simulink model "Copy_of_CM13_2024a_MachE_for_UA_HIL"  (R2024a)
settings: Solver=ode1  StartTime=0.0  StopTime=Inf  FixedStep=0.001  RelTol=1e-3  EnableMultiTasking=on
PreLoadFcn:
  | % if ~length(which('cmcmd')), cmenv; end
PostLoadFcn:
  | if any(exist('dsrtsu_mdlpostloadfcn', 'file') ~= 0), dsrtsu_mdlpostloadfcn('Execute', bdroot); end
InitFcn:
  | , if any(exist('rtifpga_mdlclblib', 'file') ~= 0), rtifpga_mdlclblib('Init', bdroot); end,
  | , if any(exist('dsmpb_private', 'file') ~= 0), dsmpb_private('dsmpb_mdlclblib', 'Init', bdroot); end,
undefined symbols (not defined in the file or in its folder): AccelCmd, ActTqLF_Nm_, ActTqLR_Nm_, ActTqRF_Nm_, ActTqRR_Nm_, BattChargeLimitMaxPwr, BattChargeLimitSocBpts, BattChargeLimitTbl, BattChrgCapcty, BattDischargeLimitSocBpts, BattDischargeLimitTbl, BattDischargeMaxPwr, BattNumCellsParallel, BattNumCellsSeries, BattOpenVoltCapBpts, BattOpenVoltTbl, BattResistSocBpts, BattResistTbl, BattResistTempBpts, BrakeMaxPrs, BrakeMaxTrq, ChassisDistCg2FrontAxle, ChassisDistCg2RearAxle, ChassisVehMass, CltchCmd, CoastDown, DecelCmd, DiffRatio, DiscIntNeverNeededParam, EnvGravCnst, EnvPrs, EnvTemp, FuelSpecificGrav, GearCmd, h, InitStates, lgSw, limitedMCT, MCT, MtrEffSpdBpts, MtrEffTbl, MtrEffTrqBpts, MtrPwrMax, MtrTrqMax, planned_speed, planned_time, pMCT, RealSimPara, ref_speed, Ref_speed, ref_time, Ref_time, rticanmm_blockfcn, rticanmm_initfcn, SteeringCmd, SupvsryCtrlRegenBrkCutOffTbl, SupvsryCtrlRegenSpdBpts, TestScnrioCycleNum, US06, VEH
libraries: simulink x264, VSIGenLib x262, etargetslib x201, dsmpblib x161, CarMaker4SL x142, rtimmsu_dsrtlib x32, vehdynlibtire x24, autolibshared x19, vehdynlibsuspension x14, vehdynlibtirecommon x14, autolibutils x10, VsrLibWheel x8
(part 9 of 47)

== system Copy_of_CM13_2024a_MachE_for_UA_HIL/CarMaker_new/IPG Vehicle/MachE CAN ==
  note: Working in Progress
  note: Gear_Shift_By_Wire_3_HS1
      | TrnGear_D_RqPt
      |
      | No_Gear
      | 0
      |
      | Park
      | 1
      |
      | Reverse
      | 2
      |
      | Neutral
      | 3
      |
      | Drive
      | 4
      |
      | Manual
      | 5
      |
      | NotUsed
      | 6
      |
      | Fault
      | 7
  note: Gear_Shift_By_Wire_HS1
      | TrnGear_D_RqDrv
      |
      | No_Gear
      | 0
      |
      | Park
      | 1
      |
      | Reverse
      | 2
      |
      | Neutral
      | 4
      |
      | Drive
      | 8
      |
      | Manual
      | 16
      |
      | Return_To_Park
      | 21/26
      |
      | Fault
      | 31
  Bus Creator : BusCreator  Inputs=6
  Bus Creator1 : BusCreator  Inputs=8
  Bus Selector : BusSelector  Commented=on  OutputSignals=Battery_Traction_2.BattTrac_U2_Actl,Battery_Traction_2.BattTrac_I2_Actl,PowertrainData_10_HS1.GearPos_D_Actl,PowertrainData_10_HS1.GearLvr_D_ActlDrv
  Bus Selector1 : BusSelector  OutputSignals=Accel_Data.VehLatLongVert_No_Cnt,Accel_Data.VehLatLongVertA_No_Cs,Accel_Data.VehVert2_A_Actl,Accel_Data.VehVertAActl_D_Qf,Accel_Data.VehLong2_A_Actl,Accel_Data.VehLongAActl_D_Qf,Accel_Data.VehLat2_A_Actl,Accel_Data.VehLatAActl_D_Qf,Yaw_Data.VehYawWActl_D_Qf,Yaw_Data.VehRolWActl_D_Qf,Yaw_Data.VehRollYaw_No_Cnt,Yaw_Data.VehRollYawW_No_Cs,Yaw_Data.VehYaw_W_Actl,Yaw_Data.VehRol_W_Actl
  Bus Selector2 : BusSelector  OutputSignals=VehLat2_A_Actl,VehLong2_A_Actl,VehVert2_A_Actl
  Bus Selector3 : BusSelector  OutputSignals=VehRol_W_Actl,VehYaw_W_Actl
  Bus Selector4 : BusSelector  OutputSignals=SteeringPinion_Data_HS2.StePinRelInit_An_Sns
  Constant : Constant  OutDataTypeStr=Inherit: Inherit via back propagation
  Constant1 : Constant  Value=0
  Gain{,1..2,6} (4 alike) : Gain  Commented=on
  Gain3 : Gain
  Gain4 : Gain
  Gain5 : Gain
  Multiport Switch : MultiPortSwitch  DataPortOrder=Zero-based contiguous  Inputs=2  zeroidx=on  SaturateOnIntegerOverflow=off  InputSameDT=off
  Multiport Switch1 : MultiPortSwitch  DataPortOrder=Zero-based contiguous  Inputs=2  zeroidx=on  SaturateOnIntegerOverflow=off  InputSameDT=off
  RTICANMM Gateway : Subsystem  InitFcn=rticanmm_initfcn(gcb, 'CANnedyGateway')  ClipboardFcn=rticanmm_blockfcn('ClipboardFcn', 'CANnedyGateway', gcb)  mask(RTICANMM){DSProperties=struct('RTI',struct('Version',uint32(1),'BlockType',struct('isSLSource',uint8(1),'isSLSink',uint8(1),'isHWSource',uint8(0),'isHWSink',uint8(0),'isSetup',uint8(0),'isInline',uint8(1),'isNonInline',uint8(0),'isInterrupt',uint8(0),'isChannelwise',uint8(0)),'IOBoardType','RTICANMM','UnitType','RTICANMM','Identifier','GATEWAY','DialogType','SL','BlockSet','RTICANMM','SlaveProcessor','CAN')), CANMMBlock=RCM_ECU, CANMMDestFolder=RTICANMM_FILES, CANMMDestBlock=RCM_Harness, CANMMProperties=struct('generaloptions',struct('gwdirection',1,'mainblksorsetups',0,'trchierarchie','','gatewayname','RCM_Gateway','mergetrc',1,'trcinclude',1,'ssOpts',struct('ssSetSampleTime','INHERITED_SAMPLE_TIME','ssSetOffsetTime','FIXED_IN_MINOR_STEP_OFFSET'),'j1939_sort_key','dir','olddirection',0),'CANGatewayID',1,'direction',struct('link',{'RCM_ECU','RCM_Harness'},'link_dbc_override',{0,0},'filesupport',{1,1},'usedirection',{true,true},'changeexcludeonline',{0,0},'excludelist',{struct('ids',{{'146','145'}},'idFormat',{{0,0}}),struct('ids',{{}},'idFormat',{{}})},'j1939',{0,0},'excludelist_j1939',{struct('id',{{}},'prio',{{}},'pdu_f',{{}},'pdu_s',{{}},'src',{{}}),struct('id',{{}},'prio',{{}},'pdu_f',{{}},'pdu_s',{{}},'src',{{}})},'data',{struct('Board','','BoardNum','','ChannelNum',''),struct('Board','','BoardNum','','ChannelNum','')},'database',{struct('FileName','RTICANMM_FILES\HS2_CAN_CX727_BEV_MY21_DCV_V21.dbc','IsRelative',1,'ClusterId',1,'ClusterList',{{'default'}}),struct('FileName','RTICANMM_FILES\HS2_CAN_CX727_BEV_MY21_DCV_V21.dbc','IsRelative',1,'ClusterId',1,'ClusterList',{{'default'}})},'FileName',{'',''},'IsRelative',{1,1},'ClusterId',{1,1},'ClusterList',{{'default'},{'default'}},'idlist',{[],[]}),'excludelist_j1939',struct('dbcsource',[],'id',{{}},'prio',{{}},'pdu_f',{{}},'pdu_s',{{}},'src',{{}}),'BlockDataVersion','4.0','directions',struct('setup',struct('source','TRC','logic','-','defaultTrc','ENABLE'),'enablematrix',struct('Direction',{['CAN Bus 1 <=> CAN Bus 2'],['CAN Bus 1  => CAN Bus 2'],['CAN Bus 1 <=  CAN Bus 2'],['CAN Bus 1  => CAN Bus 2'],['CAN Bus 1 <=  CAN Bus 2']},'Source',{'BOTH','NONE','NONE','BOTH','BOTH'},'Logic',{'OR','-','-','OR','OR'},'DefaultTrc',{'ENABLE','-','-','ENABLE','ENABLE'})),'blk',['HIL_MachE_CM10/Vehicle Under Test/Vehicle/MachE CAN/RTICANMM' char(10) 'Gateway'],'CANMMName','RCM_Gateway','TRC',struct('Name','RTICANMM_GW_RCM_Gateway_usr.trc','Path','C:\GitDev\Yunli\FordMachE\HIL-Operation\src_cm4sl\RTICANMM_FILES\RTICANMM_GW_RCM_Gateway_usr.trc','UserPath',''),'XML',struct('Name','RTICANMM_GW_RCM_Gateway.xml','Path','C:\GitDev\Yunli\FordMachE\HIL-Operation\src_cm4sl\RTICANMM_FILES\RTICANMM_GW_RCM_Gateway.xml'),'GeneratedFiles',{{'RTICANMM_GW_GW_1.c','RTICANMM_GW_GW_1.mexw64','RTICANMM_GW_GW_1.xml','RTICANMM_GW_GW_1_usr.trc','RTICANMM_GW_RCM_Gateway.c','RTICANMM_GW_RCM_Gateway.mexw64','RTICANMM_GW_RCM_Gateway.xml','RTICANMM_GW_RCM_Gateway_usr.trc'}},'allgeneratedfiles',{{'RTICANMM_GW_GW_1.c','RTICANMM_GW_GW_1.mexw64','RTICANMM_GW_GW_1.xml','RTICANMM_GW_GW_1_usr.trc','RTICANMM_GW_RCM_Gateway.c','RTICANMM_GW_RCM_Gateway.mexw64','RTICANMM_GW_RCM_Gateway.xml','RTICANMM_GW_RCM_Gateway_usr.trc'}},'version','5.3.737677.8006481482','corrsetupblks',{{['HIL_MachE_CM10/Vehicle Under Test/Vehicle/MachE CAN/RTICANMM' char(10) 'RCM_ECU'],['HIL_MachE_CM10/Vehicle Under Test/Vehicle/MachE CAN/RTICANMM' char(10) 'RCM_Harness']}},'corrsetupids',{{'RCM_ECU';'RCM_Harness'}},'UserTraceMerged','off','MMType','RTICANMM'), CANMMType=CANnedyGateway}
      settings: AttributesFormatString=RCM_ECU <=> RCM_Harness  CopyFcn=rticanmm_blockfcn('CopyFcn', 'CANnedyGateway', gcb)  DeleteFcn=rticanmm_blockfcn('DeleteFcn', 'CANnedyGateway', gcb)  ModelCloseFcn=rticanmm_blockfcn('ModelCloseFcn', 'CANnedyGateway', gcb)  NameChangeFcn=rticanmm_blockfcn('NameChangeFcn', 'CANnedyGateway', gcb)  OpenFcn=try, rticanmm_gw_gui('create',gcb); ; catch,errordlg({lasterr, '','Please check your RTI installation.'},['Error: ' upper(bdroot)], 'replace'); end  MoveFcn=rticanmm_blockfcn('MoveFcn', 'CANnedyGateway', gcb)
      mask Help: eval('rticanmm_quickstart(''create'', gcb);', 'disp(lasterr);')
      mask Display:
      | disp(sprintf(['RTI CAN\nMultiMessage\nGateway']))
      | port_label('input',1,'Enable')
      | port_label('output',1,'Bus1TXCounter')
      | port_label('output',2,'Bus1RXCounter')
      | port_label('output',3,'Bus2TXCounter')
      | port_label('output',4,'Bus2RXCounter')
  RTICANMM GeneralSetup : Subsystem  InitFcn=rticanmm_initfcn(gcb, 'CANnedySettings')  ClipboardFcn=rticanmm_blockfcn('ClipboardFcn', 'CANnedySettings', gcb)  mask(RTICANMM){DSProperties=struct('RTI',struct('Version',uint32(1),'BlockType',struct('isSLSource',uint8(1),'isSLSink',uint8(1),'isHWSource',uint8(0),'isHWSink',uint8(0),'isSetup',uint8(0),'isInline',uint8(1),'isNonInline',uint8(0),'isInterrupt',uint8(0),'isChannelwise',uint8(0)),'IOBoardType','RTICANMM','UnitType','RTICANMM','Identifier','GENERALSETUP','DialogType','SL','BlockSet','RTICANMM','SlaveProcessor','CAN')), CANMMDestFolder=RTICANMM_FILES, CANMMBuildDir=., CANMMAddPaths=on, CANMMAddpathUserMake=on, CANMMRemovePathOnclose=on, CANMMType=CANnedySettings, CANMMProperties=struct('modelroot','C:\CM_Projects\UA_cave\CM13_proj\src_cm4dspace_realsim','generalsettings',struct('filesettings',struct('destfolder',struct('Name','RTICANMM_FILES','Check',1),'buildfolder',struct('Name','.','Check',1),'AbsDestfolder',struct('Name','C:\CM_Projects\UA_cave\CM13_proj\src_cm4dspace_realsim\RTICANMM_FILES'),'AbsBuildfolder',struct('Name','C:\CM_Projects\UA_cave\CM13_proj\src_cm4dspace_realsim'))),'options',struct('addpaths',1,'rmpaths',1,'addtrcexclusion',true,'cannavigator',struct('checkmonitoring',0),'show_usrtrc',0,'use_usrtrc',0,'addpath2usrmk',1),'advanced',struct('options',ones(1,100)),'MPSetup',{{}},'modelname','CM13_2024a_MachE','blockdata',struct('generalsettings',struct('filesettings',struct('destfolder',struct('Name','.','Check',1),'AbsDestfolder',struct('Name','T:\TOOL_SOURCES\CANnedy\m'),'buildfolder',struct('Name','.','Check',1),'AbsBuildfolder',struct('Name','C:\MATLAB6p5\work'))),'options',struct('addpaths',1,'rmpaths',1,'addpath2usrmk',1),'modelname','rticanmmlib','modelroot','T:\TOOL_SOURCES\CANnedy\m'),'MMType','RTICANMM','block',['CM13_2024a_MachE/CarMaker/IPG Vehicle/MachE CAN/RTICANMM' char(10) 'GeneralSetup'],'RTI',struct('Type','DSRT','Ver','24.1','Date','02-May-2024'),'version','24.1.739338.0305092592','userdata',struct('HostServiceChannelID',{{'MachE_FD1','RCM_ECU','RCM_Harness','MachE_HS1',[]}}))}
      mask prompts: CANMMDestFolder "Destination Folder for generated Files:"; CANMMBuildDir "Build Directory (*_usr.mk, *_usr.trc)"; CANMMAddPaths "Add Paths automatically"; CANMMAddpathUserMake "Add Paths to UserMake-File"; CANMMRemovePathOnclose "Remove added Path on ModelClose"
      mask init:
      | rticanmm_initfcn(gcb,'CANnedyGeneralSettings')
      settings: CopyFcn=rticanmm_blockfcn('CopyFcn', 'CANnedySettings', gcb)  DeleteFcn=rticanmm_blockfcn('DeleteFcn', 'CANnedySettings', gcb)  ModelCloseFcn=rticanmm_blockfcn('CloseFcn', 'CANnedyGeneralSettings', gcb)  NameChangeFcn=rticanmm_blockfcn('NameChangeFcn', 'CANnedySettings', gcb)  OpenFcn=try, rticanmm_gs_gui('create',gcb), ; catch,errordlg({lasterr, '','Please check your RTI installation.'},['Error: ' upper(bdroot)], 'replace'); end  MoveFcn=rticanmm_blockfcn('MoveFcn', 'CANnedySettings', gcb)
      mask Help: try, rticanmm_quickstart('create', gcb); catch ME, disp(ME.message);end
      mask Display: disp(sprintf(['RTI CAN\nMultiMessage\nGeneralSetup']))
  RTICANMM MachE_HS1 : Subsystem  InitFcn=rticanmm_blockfcn('InitFcn', 'CANnedySetup', gcb)  ClipboardFcn=rticanmm_blockfcn('ClipboardFcn', 'CANnedySetup', gcb)  mask(RTICANMM){DSProperties=struct('RTI',struct('Version',uint32(1),'BlockType',struct('isSLSource',uint8(1),'isSLSink',uint8(1),'isHWSource',uint8(0),'isHWSink',uint8(0),'isSetup',uint8(0),'isInline',uint8(1),'isNonInline',uint8(0),'isInterrupt',uint8(0),'isChannelwise',uint8(0)),'IOBoardType','RTICANMM','UnitType','RTICANMM','Identifier','BUSSETUP','DialogType','SL','BlockSet','RTICANMM','SlaveProcessor','CAN')), CANMMProperties=struct('cannedy',struct('data',struct('options',struct('controllername','MachE_HS1','controllernameautomatic',0,'loglevel','0','checkrealtime',0,'checkchangebaudrate',0,'sampletime','1.000','CANControllerStatus',0,'NumberofStuffErr',0,'NumberofFormErr',0,'NumberofAckErr',0,'NumberofBit0Err',0,'NumberofsuccrecRX',0,'Numberofsuccsent',0,'NumberofBit1Err',0,'NumberofCRCErr',0,'NumberoflostRX',0,'Busoff',0,'Busload',0,'OperationPending',0,'TxRetryCount',3,'addtrcexclusion',true,'cannavigator',struct('checkmonitoring',0,'checkinternmonitoring',0),'show_usrtrc',0,'use_usrtrc',0,'checkchangebaudrateFD',0,'errorframegeneration',0,'efgenabled',1),'modelroot','C:\CM_Projects\UA_cave\CM11_proj\src_cm4sl_ds','generalsettings',struct('setupdata',struct('board','DS2671','boardno',1,'channelno',1,'Type','STD','transceiver',['ISO 11898-2 HIGH SPEED CAN'],'busconfig',[],'feedthrough','false','resistance',struct('r120',1,'roff',0,'r16',1,'r10',0),'baudrate','500','Frequency',[24 36],'samplemode',1,'commChannelTJA1041',6,'config',struct('standard',1,'advanced',0,'register',struct('btr0','0xC0','btr1','0x6F','sp','70','sjw','v','tseg1','15','tseg2','6','brp','0','smpl','0','btr0_36','0x1','btr1_36','0x2D','sp_36','83','sjw_36','0','tseg1_36','12','tseg2_36','2','brp_36','1','smpl_36','0','btr0_64','0x3','btr1_64','0x2B','sp_64','81','sjw_64','0','tseg1_64','11','tseg2_64','2','brp_64','3','smpl_64','0')),'channelcfg',struct('INTENDISABLE','CAN_INT_DISABLE','intenable',0),'SETUPID','RTICANMM_MachE_HS1_ID','CONTROLLER_ID','CANMM_CTL_SETUP_MachE_HS1','mainblock_includefile','RTICANMM_SETUP_MachE_HS1','canfdenable',0,'canfdboardselected',1,'slotno',1,'moduletype','DS4342','baudrateFD','4000','samplePoint','80','samplePointFD','80','termination','TERMINATION_ON'),'filesettings',struct('destfolder',struct('Name','RTICANMM_FILES','Check',1),'buildfolder',struct('Name','.','Check',1))),'advanced',struct('options',ones(1,100)),'partialnetdata',struct('switchedon',0,'format','STD','idmask',['XXXXX XXXXXXXX XXXXXXXX XXXXXXXX'],'idcode','0','idfilter','0','datamaskused',0,'datalength','0','datamask','0x0000000000000000','partialnetworkenable',0)),'blk',['RS_DS_CM11_noSimulinkRS_FordTopology/CarMaker/IPG Vehicle/MachE CAN/RTICANMM' char(10) 'MachE_HS1'],'allgeneratedfiles',{{'C:\CM_Projects\UA_cave\CM11_proj\src_cm4sl_ds\RTICANMM_FILES\RTICANMM_SETUP_Bat_monitor.c','C:\CM_Projects\UA_cave\CM11_proj\src_cm4sl_ds\RTICANMM_FILES\RTICANMM_SETUP_Bat_monitor.h','C:\CM_Projects\UA_cave\CM11_proj\src_cm4sl_ds\RTICANMM_FILES\RTICANMM_SETUP_CAN_BAT.c','C:\CM_Projects\UA_cave\CM11_proj\src_cm4sl_ds\RTICANMM_FILES\RTICANMM_SETUP_CAN_BAT.h','C:\CM_Projects\UA_cave\CM11_proj\src_cm4sl_ds\RTICANMM_FILES\RTICANMM_SETUP_MachE_HS1.c','C:\CM_Projects\UA_cave\CM11_proj\src_cm4sl_ds\RTICANMM_FILES\RTICANMM_SETUP_MachE_HS1.h','c:\cm_projects\ua_cave\cm11_proj\src_cm4sl_ds\rticanmm_files\rticanmm_setup_bat_monitor.mexw64','c:\cm_projects\ua_cave\cm11_proj\src_cm4sl_ds\rticanmm_files\rticanmm_setup_can_bat.mexw64','c:\cm_projects\ua_cave\cm11_proj\src_cm4sl_ds\rticanmm_files\rticanmm_setup_mache_hs1.mexw64'}},'ismp',false,'BlockDataVersion','0.9.0','recreate',0,'CANnedyTag','MachE_HS1'),'CANnedynew',0,'CANnedySettings','MachE_HS1','GeneratedFiles',{{'C:\CM_Projects\UA_cave\CM11_proj\src_cm4sl_ds\RTICANMM_FILES\RTICANMM_SETUP_Bat_monitor.c','C:\CM_Projects\UA_cave\CM11_proj\src_cm4sl_ds\RTICANMM_FILES\RTICANMM_SETUP_Bat_monitor.h','C:\CM_Projects\UA_cave\CM11_proj\src_cm4sl_ds\RTICANMM_FILES\RTICANMM_SETUP_CAN_BAT.c','C:\CM_Projects\UA_cave\CM11_proj\src_cm4sl_ds\RTICANMM_FILES\RTICANMM_SETUP_CAN_BAT.h','C:\CM_Projects\UA_cave\CM11_proj\src_cm4sl_ds\RTICANMM_FILES\RTICANMM_SETUP_MachE_HS1.c','C:\CM_Projects\UA_cave\CM11_proj\src_cm4sl_ds\RTICANMM_FILES\RTICANMM_SETUP_MachE_HS1.h','c:\cm_projects\ua_cave\cm11_proj\src_cm4sl_ds\rticanmm_files\rticanmm_setup_bat_monitor.mexw64','c:\cm_projects\ua_cave\cm11_proj\src_cm4sl_ds\rticanmm_files\rticanmm_setup_can_bat.mexw64','c:\cm_projects\ua_cave\cm11_proj\src_cm4sl_ds\rticanmm_files\rticanmm_setup_mache_hs1.mexw64'}},'SFCN','RTICANMM_SETUP_MachE_HS1.c','HostService',struct('Tags',struct('DATA','RTICANMM_MonitorData','TimeStampGlobal','RTICANMM_MonitoringTimeStamp','TimeStampGlobalEnable','RTICANMM_MonitoringTimeStampEnable','Enable','CANMMMonitor_MachE_HS1','TimeStamp','MonitoringTimeStamp_MachE_HS1'),'DATA',struct('Length',18),'Info',struct('Desc',{'ID','Service','Data1','Data2','Data3','Data4','Data5','Data6','Data7','Data8','Data9','Data10','Data11','Data12','Data13','Data14','Data15','Data16'}),'Names',struct('TimeStampGlobal','TimeStamp','TimeStampGlobalEnable','TimeStamp_Enable','Enable','Monitoring_Enable','TimeStamp','Monitoring_TimeStamp'),'ChannelID',4)), CANMMType=CANnedySetup, CANMMFolder=C:\CM_Projects\UA_cave\CM13_proj\src_cm4dspace_realsim, CANMMDestFolder=RTICANMM_FILES, CANMMSettings=MachE_HS1, CANMMSFcn=RTICANMM_SETUP_MachE_HS1, CANMMBoard=DS2671, CANMMBoardNum=1, CANMMChannel=1}
      settings: AttributesFormatString=%<CANMMSettings>  CopyFcn=rticanmm_blockfcn('CopyFcn', 'CANnedySetup', gcb)  DeleteFcn=rticanmm_blockfcn('DeleteFcn', 'CANnedySetup', gcb)  ModelCloseFcn=rticanmm_blockfcn('ModelCloseFcn', 'CANnedySetup', gcb)  NameChangeFcn=rticanmm_blockfcn('NameChangeFcn', 'CANnedySetup', gcb)  OpenFcn=try, rticanmm_setup_gui('create',gcb); ; catch,errordlg({lasterr, '','Please check your RTI installation.'},['Error: ' upper(bdroot)], 'replace'); end  MoveFcn=rticanmm_blockfcn('MoveFcn', 'CANnedySetup', gcb)
      mask Help: try, rticanmm_quickstart('create', gcb); catch ME, disp(ME.message);end
      mask Display:
      | disp('RTI CAN\nMultiMessage\nControllerSetup')
      | 
      | port_label('input', 1 , 'Variation')
      | port_label('input', 2 , 'Reset')
  RTICANMM MachE_HS2 : dsmpblib/Data Outport  Priority=-10000  Commented=on
      settings: SourceProductName=dSPACE Model Interface Package for Simulink (MIPS)
  RTICANMM MainBlock : Subsystem  InitFcn=rticanmm_blockfcn('InitFcn', 'CANnedy', gcb)  ClipboardFcn=rticanmm_blockfcn('ClipboardFcn', 'CANnedy', gcb)  mask(RTICANMM){DSProperties=struct('RTI',struct('Version',uint32(1),'BlockType',struct('isSLSource',uint8(1),'isSLSink',uint8(1),'isHWSource',uint8(0),'isHWSink',uint8(0),'isSetup',uint8(0),'isInline',uint8(1),'isNonInline',uint8(0),'isInterrupt',uint8(0),'isChannelwise',uint8(0)),'IOBoardType','RTICANMM','UnitType','RTICANMM','Identifier','Mainblock','DialogType','SL','BlockSet','RTICANMM','SlaveProcessor','CAN')), CANMMProperties=struct('RTICANMMVersion','24.1','RTICANMMVersionIntern','24.1.739338.0305092592','RTICANMMDate','02-May-2024','Settings','RTICANMM_MAIN_RCM_ECU','UserTracePath','','ModelPath','C:\CM_Projects\UA_cave\CM13_proj\src_cm4dspace_realsim','filesettings',struct('FileName','RTICANMM_FILES\HS2_CAN_CX727_BEV_MY21_DCV_V21.dbc','IsRelative',1,'ClusterId',1,'ClusterList',{{'default'}},'destfolder',struct('Name','RTICANMM_FILES','Check',1),'buildfolder',struct('Name','.','Check',1),'onlyfreerawcapture',0,'overlapping2variant',0,'canfdsupport',0,'shortestJ2container',1),'onlyfreerawcapture',0,'Board','DS2671','BoardNum','1','ChannelNum','1','Variation','1','SetupId','RCM_ECU','MARK',['3F3F0BA07D5203DDC276938B2E5007';'05A5443C266C0D2A8F1F40D5383B99';'71789265470E2889516AD636A12D58';'133F6E799A646EEE8C7A8443A0E6AF';'583ADA83977C34593CB39FD6B3AB52'],'date','08-May-2025','clock',['08.05.2025 17:21:14'],'recreate',0,'RTIVER','DSRT','j1939',0,'TRC',struct('include',1),'rtsupport',struct('XMLFile','C:\CM_Projects\UA_cave\CM13_proj\src_cm4dspace_realsim\RTICANMM_FILES\RTICANMM_MAIN_RCM_ECU.xml','DBCXML',struct('Path','C:\CM_Projects\UA_cave\CM13_proj\src_cm4dspace_realsim\RTICANMM_FILES\RTICANMM_MAIN_RCM_ECU_dbc.xml','support',1,'Name','HS2_CAN_CX727_BEV_MY21_DCV_V21.dbc','Date',['28-Mar-2023 17:18:35'],'Type','mixed','DBCSupport','ON'))), CANMMType=CANnedy, CANMMUserTraceMerged=off, CANMMUserTracePath=, CANMMChannelNum=1, CANMMBoardNum=1, CANMMDestFolder=RTICANMM_FILES, CANMMFolder=., CANMMSetupId=RCM_ECU, CANMMsave2mat=['3F3F0BA07D5203DDC276938B2E5007';'05A5443C266C0D2A8F1F40D5383B99';'71789265470E2889516AD636A12D58';'133F6E799A646EEE8C7A8443A0E6AF';'583ADA83977C34593CB39FD6B3AB52'], CANMMName=RCM_ECU, CANMMSettings=RTICANMM_MAIN_RCM_ECU, CANMMIntermediateTag=RTICANMM_MAIN_RCM_ECU_intermediate, CANMMsfcnname=RTICANMM_MAIN_RCM_ECU}
      mask init:
      | rticanmm_initfcn(gcb, CANMMType, CANMMsfcnname)
      settings: AttributesFormatString=RCM_ECU[RCM_ECU]  CopyFcn=rticanmm_blockfcn('CopyFcn', 'CANnedy', gcb)  DeleteFcn=rticanmm_blockfcn('DeleteFcn', 'CANnedy', gcb)  ModelCloseFcn=rticanmm_blockfcn('ModelCloseFcn', 'CANnedy', gcb)  NameChangeFcn=rticanmm_blockfcn('NameChangeFcn', 'CANnedy', gcb)  OpenFcn=try, rticanmm_main_gui('create',gcb); ; catch,errordlg({lasterr, '','Please check your RTI installation.'},['Error: ' upper(bdroot)], 'replace'); end  MoveFcn=rticanmm_blockfcn('MoveFcn', 'CANnedy', gcb)
      mask Help: try, rticanmm_quickstart('create', gcb); catch ME, disp(ME.message);end
      mask Display:
      | disp(sprintf('RTI CAN\nMultiMessage\nMainBlock'))
      | port_label('output', 1, 'RX Data')
  RTICANMM MainBlock1 : Subsystem  InitFcn=rticanmm_blockfcn('InitFcn', 'CANnedy', gcb)  ClipboardFcn=rticanmm_blockfcn('ClipboardFcn', 'CANnedy', gcb)  mask(RTICANMM){DSProperties=struct('RTI',struct('Version',uint32(1),'BlockType',struct('isSLSource',uint8(1),'isSLSink',uint8(1),'isHWSource',uint8(0),'isHWSink',uint8(0),'isSetup',uint8(0),'isInline',uint8(1),'isNonInline',uint8(0),'isInterrupt',uint8(0),'isChannelwise',uint8(0)),'IOBoardType','RTICANMM','UnitType','RTICANMM','Identifier','Mainblock','DialogType','SL','BlockSet','RTICANMM','SlaveProcessor','CAN')), CANMMProperties=struct('RTICANMMVersion','24.1','RTICANMMVersionIntern','24.1.739338.0305092592','RTICANMMDate','02-May-2024','Settings','RTICANMM_MAIN_RCM_Harness','UserTracePath','','ModelPath','C:\CM_Projects\UA_cave\CM13_proj\src_cm4dspace_realsim','filesettings',struct('FileName','RTICANMM_FILES\HS2_CAN_CX727_BEV_MY21_DCV_V21.dbc','IsRelative',1,'ClusterId',1,'ClusterList',{{'default'}},'destfolder',struct('Name','RTICANMM_FILES','Check',1),'buildfolder',struct('Name','.','Check',1),'onlyfreerawcapture',0,'overlapping2variant',0,'canfdsupport',0,'shortestJ2container',1),'onlyfreerawcapture',0,'Board','DS2671','BoardNum','1','ChannelNum','1','Variation','1','SetupId','RCM_Harness','MARK',['0E503861171A6E489AB1727A1B00A0';'5B089505471349A0989225D608F478';'A09B19290F681933AA09BB18006871';'A77AEF5BA06E247EAF11AAF4437957';'95560815972E75D997A4373D234FA8'],'date','08-May-2025','clock',['08.05.2025 17:03:06'],'recreate',0,'RTIVER','DSRT','j1939',0,'TRC',struct('include',1),'rtsupport',struct('XMLFile','C:\CM_Projects\UA_cave\CM13_proj\src_cm4dspace_realsim\RTICANMM_FILES\RTICANMM_MAIN_RCM_Harness.xml','DBCXML',struct('Path','C:\CM_Projects\UA_cave\CM13_proj\src_cm4dspace_realsim\RTICANMM_FILES\RTICANMM_MAIN_RCM_Harness_dbc.xml','support',1,'Name','HS2_CAN_CX727_BEV_MY21_DCV_V21.dbc','Date',['28-Mar-2023 17:18:35'],'Type','mixed','DBCSupport','ON'))), CANMMType=CANnedy, CANMMUserTraceMerged=off, CANMMUserTracePath=, CANMMChannelNum=1, CANMMBoardNum=1, CANMMDestFolder=RTICANMM_FILES, CANMMFolder=., CANMMSetupId=RCM_Harness, CANMMsave2mat=['0E503861171A6E489AB1727A1B00A0';'5B089505471349A0989225D608F478';'A09B19290F681933AA09BB18006871';'A77AEF5BA06E247EAF11AAF4437957';'95560815972E75D997A4373D234FA8'], CANMMName=RCM_Harness, CANMMSettings=RTICANMM_MAIN_RCM_Harness, CANMMIntermediateTag=RTICANMM_MAIN_RCM_Harness_intermediate, CANMMsfcnname=RTICANMM_MAIN_RCM_Harness}
      mask init:
      | rticanmm_initfcn(gcb, CANMMType, CANMMsfcnname)
      settings: AttributesFormatString=RCM_Harness[RCM_Harness]  CopyFcn=rticanmm_blockfcn('CopyFcn', 'CANnedy', gcb)  DeleteFcn=rticanmm_blockfcn('DeleteFcn', 'CANnedy', gcb)  ModelCloseFcn=rticanmm_blockfcn('ModelCloseFcn', 'CANnedy', gcb)  NameChangeFcn=rticanmm_blockfcn('NameChangeFcn', 'CANnedy', gcb)  OpenFcn=try, rticanmm_main_gui('create',gcb); ; catch,errordlg({lasterr, '','Please check your RTI installation.'},['Error: ' upper(bdroot)], 'replace'); end  MoveFcn=rticanmm_blockfcn('MoveFcn', 'CANnedy', gcb)
      mask Help: try, rticanmm_quickstart('create', gcb); catch ME, disp(ME.message);end
      mask Display:
      | disp(sprintf('RTI CAN\nMultiMessage\nMainBlock'))
      | port_label('input', 1, 'TX Data')
      | port_label('output', 1, 'RX Data')
  RTICANMM MainBlock2 : Subsystem  Commented=on  InitFcn=rticanmm_blockfcn('InitFcn', 'CANnedy', gcb)  ClipboardFcn=rticanmm_blockfcn('ClipboardFcn', 'CANnedy', gcb)  mask(RTICANMM){DSProperties=struct('RTI',struct('Version',uint32(1),'BlockType',struct('isSLSource',uint8(1),'isSLSink',uint8(1),'isHWSource',uint8(0),'isHWSink',uint8(0),'isSetup',uint8(0),'isInline',uint8(1),'isNonInline',uint8(0),'isInterrupt',uint8(0),'isChannelwise',uint8(0)),'IOBoardType','RTICANMM','UnitType','RTICANMM','Identifier','Mainblock','DialogType','SL','BlockSet','RTICANMM','SlaveProcessor','CAN')), CANMMProperties=struct('RTICANMMVersion','5.7','RTICANMMVersionIntern','5.7.738421.7765740741','RTICANMMDate','02-Nov-2021','Settings','RTICANMM_MAIN_MachE_HS1','UserTracePath','','ModelPath','C:\CM_Projects\UA_cave\CM11_proj\src_cm4sl_ds','filesettings',struct('FileName','RTICANMM_FILES\HS1_CAN_CX727_BEV_MY21_DCV_V21.dbc','IsRelative',1,'ClusterId',1,'ClusterList',{{'default'}},'destfolder',struct('Name','RTICANMM_FILES','Check',1),'buildfolder',struct('Name','.','Check',1),'onlyfreerawcapture',0,'overlapping2variant',0,'canfdsupport',0,'shortestJ2container',1),'onlyfreerawcapture',0,'Board','DS2671','BoardNum','1','ChannelNum','1','Variation','1','SetupId','MachE_HS1','MARK',['20CBE71203884C91FC0BDF2386A725';'1376ED9E18623D415299BF6987B2BF';'0012B29A86D3424CBD8951AC432984';'B479623848823C255B19C6499B8B7F';'B300B99E5D56920EA3297C7D0176F1'],'date','19-Sep-2024','clock',['19.09.2024 17:17:45'],'recreate',0,'RTIVER','DSRT','j1939',0,'TRC',struct('include',1),'rtsupport',struct('XMLFile','C:\CM_Projects\UA_cave\CM11_proj\src_cm4sl_ds\RTICANMM_FILES\RTICANMM_MAIN_MachE_HS1.xml','DBCXML',struct('Path','C:\CM_Projects\UA_cave\CM11_proj\src_cm4sl_ds\RTICANMM_FILES\RTICANMM_MAIN_MachE_HS1_dbc.xml','support',1,'Name','HS1_CAN_CX727_BEV_MY21_DCV_V21.dbc','Date',['28-Mar-2023 17:18:35'],'Type','mixed','DBCSupport','ON'))), CANMMType=CANnedy, CANMMUserTraceMerged=off, CANMMUserTracePath=, CANMMChannelNum=1, CANMMBoardNum=1, CANMMDestFolder=RTICANMM_FILES, CANMMFolder=., CANMMSetupId=MachE_HS1, CANMMsave2mat=['20CBE71203884C91FC0BDF2386A725';'1376ED9E18623D415299BF6987B2BF';'0012B29A86D3424CBD8951AC432984';'B479623848823C255B19C6499B8B7F';'B300B99E5D56920EA3297C7D0176F1'], CANMMName=MachE_HS1, CANMMSettings=RTICANMM_MAIN_MachE_HS1, CANMMIntermediateTag=RTICANMM_MAIN_MachE_HS1_intermediate, CANMMsfcnname=RTICANMM_MAIN_MachE_HS1}
      mask init:
      | rticanmm_initfcn(gcb, CANMMType, CANMMsfcnname)
      settings: AttributesFormatString=MachE_HS1[MachE_HS1]  CopyFcn=rticanmm_blockfcn('CopyFcn', 'CANnedy', gcb)  DeleteFcn=rticanmm_blockfcn('DeleteFcn', 'CANnedy', gcb)  ModelCloseFcn=rticanmm_blockfcn('ModelCloseFcn', 'CANnedy', gcb)  NameChangeFcn=rticanmm_blockfcn('NameChangeFcn', 'CANnedy', gcb)  OpenFcn=try, rticanmm_main_gui('create',gcb); ; catch,errordlg({lasterr, '','Please check your RTI installation.'},['Error: ' upper(bdroot)], 'replace'); end  MoveFcn=rticanmm_blockfcn('MoveFcn', 'CANnedy', gcb)
      mask Help: try, rticanmm_quickstart('create', gcb); catch ME, disp(ME.message);end
      mask Display:
      | disp(sprintf('RTI CAN\nMultiMessage\nMainBlock'))
      | port_label('input', 1, 'TX Data')
  RTICANMM RCM_ECU : Subsystem  InitFcn=rticanmm_blockfcn('InitFcn', 'CANnedySetup', gcb)  ClipboardFcn=rticanmm_blockfcn('ClipboardFcn', 'CANnedySetup', gcb)  mask(RTICANMM){DSProperties=struct('RTI',struct('Version',uint32(1),'BlockType',struct('isSLSource',uint8(1),'isSLSink',uint8(1),'isHWSource',uint8(0),'isHWSink',uint8(0),'isSetup',uint8(0),'isInline',uint8(1),'isNonInline',uint8(0),'isInterrupt',uint8(0),'isChannelwise',uint8(0)),'IOBoardType','RTICANMM','UnitType','RTICANMM','Identifier','BUSSETUP','DialogType','SL','BlockSet','RTICANMM','SlaveProcessor','CAN')), CANMMProperties=struct('cannedy',struct('data',struct('options',struct('controllername','RCM_ECU','controllernameautomatic',0,'loglevel','0','checkrealtime',0,'checkchangebaudrate',0,'sampletime','1.000','CANControllerStatus',0,'NumberofStuffErr',0,'NumberofFormErr',0,'NumberofAckErr',0,'NumberofBit0Err',0,'NumberofsuccrecRX',0,'Numberofsuccsent',0,'NumberofBit1Err',0,'NumberofCRCErr',0,'NumberoflostRX',0,'Busoff',0,'Busload',0,'OperationPending',0,'TxRetryCount',3,'addtrcexclusion',true,'cannavigator',struct('checkmonitoring',0,'checkinternmonitoring',0),'show_usrtrc',0,'use_usrtrc',0,'checkchangebaudrateFD',0,'errorframegeneration',0,'efgenabled',1),'modelroot','C:\GitDev\Yunli\FordMachE\HIL-Operation\src_cm4sl','generalsettings',struct('setupdata',struct('board','DS2671','boardno',1,'channelno',1,'Type','STD','transceiver',['ISO 11898-2 HIGH SPEED CAN'],'busconfig',[],'feedthrough','false','resistance',struct('r120',1,'roff',0,'r16',1,'r10',0),'baudrate','500','Frequency',[24 36],'samplemode',1,'commChannelTJA1041',6,'config',struct('standard',1,'advanced',0,'register',struct('btr0','0xC0','btr1','0x6F','sp','70','sjw','v','tseg1','15','tseg2','6','brp','0','smpl','0','btr0_36','0x1','btr1_36','0x2D','sp_36','83','sjw_36','0','tseg1_36','12','tseg2_36','2','brp_36','1','smpl_36','0','btr0_64','0x3','btr1_64','0x2B','sp_64','81','sjw_64','0','tseg1_64','11','tseg2_64','2','brp_64','3','smpl_64','0')),'channelcfg',struct('INTENDISABLE','CAN_INT_DISABLE','intenable',0),'SETUPID','RTICANMM_RCM_ECU_ID','CONTROLLER_ID','CANMM_CTL_SETUP_RCM_ECU','mainblock_includefile','RTICANMM_SETUP_RCM_ECU','canfdenable',0,'canfdboardselected',1,'slotno',1,'moduletype','DS4342','baudrateFD','2000','samplePoint','80','samplePointFD','80','termination','TERMINATION_ON'),'filesettings',struct('destfolder',struct('Name','RTICANMM_FILES','Check',1),'buildfolder',struct('Name','.','Check',1))),'advanced',struct('options',ones(1,100)),'partialnetdata',struct('switchedon',0,'format','STD','idmask',['XXXXX XXXXXXXX XXXXXXXX XXXXXXXX'],'idcode','0','idfilter','0','datamaskused',0,'datalength','0','datamask','0x0000000000000000','partialnetworkenable',0)),'blk',['HIL_MachE_CM10/Vehicle Under Test/Vehicle/AEB Flag/RTICANMM' char(10) 'ControllerSetup1'],'allgeneratedfiles',{{'C:\GitDev\Yunli\FordMachE\HIL-Operation\src_cm4sl\RTICANMM_FILES\RTICANMM_SETUP_RCM_ECU.c','C:\GitDev\Yunli\FordMachE\HIL-Operation\src_cm4sl\RTICANMM_FILES\RTICANMM_SETUP_RCM_ECU.h','C:\GitDev\Yunli\FordMachE\HIL-Operation\src_cm4sl\RTICANMM_FILES\RTICANMM_SETUP_RCM_Harness.c','C:\GitDev\Yunli\FordMachE\HIL-Operation\src_cm4sl\RTICANMM_FILES\RTICANMM_SETUP_RCM_Harness.h','c:\gitdev\yunli\fordmache\hil-operation\src_cm4sl\rticanmm_files\rticanmm_setup_rcm_ecu.mexw64','c:\gitdev\yunli\fordmache\hil-operation\src_cm4sl\rticanmm_files\rticanmm_setup_rcm_harness.mexw64'}},'ismp',false,'BlockDataVersion','0.9.0','recreate',0,'CANnedyTag','RCM_ECU'),'CANnedynew',0,'CANnedySettings','RCM_ECU','GeneratedFiles',{{'C:\GitDev\Yunli\FordMachE\HIL-Operation\src_cm4sl\RTICANMM_FILES\RTICANMM_SETUP_RCM_ECU.c','C:\GitDev\Yunli\FordMachE\HIL-Operation\src_cm4sl\RTICANMM_FILES\RTICANMM_SETUP_RCM_ECU.h','C:\GitDev\Yunli\FordMachE\HIL-Operation\src_cm4sl\RTICANMM_FILES\RTICANMM_SETUP_RCM_Harness.c','C:\GitDev\Yunli\FordMachE\HIL-Operation\src_cm4sl\RTICANMM_FILES\RTICANMM_SETUP_RCM_Harness.h','c:\gitdev\yunli\fordmache\hil-operation\src_cm4sl\rticanmm_files\rticanmm_setup_rcm_ecu.mexw64','c:\gitdev\yunli\fordmache\hil-operation\src_cm4sl\rticanmm_files\rticanmm_setup_rcm_harness.mexw64'}},'SFCN','RTICANMM_SETUP_RCM_ECU.c','HostService',struct('Tags',struct('DATA','RTICANMM_MonitorData','TimeStampGlobal','RTICANMM_MonitoringTimeStamp','TimeStampGlobalEnable','RTICANMM_MonitoringTimeStampEnable','Enable','CANMMMonitor_RCM_ECU','TimeStamp','MonitoringTimeStamp_RCM_ECU'),'DATA',struct('Length',18),'Info',struct('Desc',{'ID','Service','Data1','Data2','Data3','Data4','Data5','Data6','Data7','Data8','Data9','Data10','Data11','Data12','Data13','Data14','Data15','Data16'}),'Names',struct('TimeStampGlobal','TimeStamp','TimeStampGlobalEnable','TimeStamp_Enable','Enable','Monitoring_Enable','TimeStamp','Monitoring_TimeStamp'),'ChannelID',4)), CANMMType=CANnedySetup, CANMMFolder=C:\CM_Projects\UA_cave\CM13_proj\src_cm4dspace_realsim, CANMMDestFolder=RTICANMM_FILES, CANMMSettings=RCM_ECU, CANMMSFcn=RTICANMM_SETUP_RCM_ECU, CANMMBoard=DS2671, CANMMBoardNum=1, CANMMChannel=1}
      settings: AttributesFormatString=%<CANMMSettings>  CopyFcn=rticanmm_blockfcn('CopyFcn', 'CANnedySetup', gcb)  DeleteFcn=rticanmm_blockfcn('DeleteFcn', 'CANnedySetup', gcb)  ModelCloseFcn=rticanmm_blockfcn('ModelCloseFcn', 'CANnedySetup', gcb)  NameChangeFcn=rticanmm_blockfcn('NameChangeFcn', 'CANnedySetup', gcb)  OpenFcn=try, rticanmm_setup_gui('create',gcb); ; catch,errordlg({lasterr, '','Please check your RTI installation.'},['Error: ' upper(bdroot)], 'replace'); end  MoveFcn=rticanmm_blockfcn('MoveFcn', 'CANnedySetup', gcb)
      mask Help: eval('rticanmm_quickstart(''create'', gcb);', 'disp(lasterr);')
      mask Display:
      | disp('RTI CAN\nMultiMessage\nControllerSetup')
      | 
      | port_label('input', 1 , 'Variation')
      | port_label('input', 2 , 'Reset')
  RTICANMM RCM_ECU1 : dsmpblib/Data Outport  Priority=-10000  Commented=on
      settings: SourceProductName=dSPACE Model Interface Package for Simulink (MIPS)
  RTICANMM RCM_Harness : Subsystem  InitFcn=rticanmm_blockfcn('InitFcn', 'CANnedySetup', gcb)  ClipboardFcn=rticanmm_blockfcn('ClipboardFcn', 'CANnedySetup', gcb)  mask(RTICANMM){DSProperties=struct('RTI',struct('Version',uint32(1),'BlockType',struct('isSLSource',uint8(1),'isSLSink',uint8(1),'isHWSource',uint8(0),'isHWSink',uint8(0),'isSetup',uint8(0),'isInline',uint8(1),'isNonInline',uint8(0),'isInterrupt',uint8(0),'isChannelwise',uint8(0)),'IOBoardType','RTICANMM','UnitType','RTICANMM','Identifier','BUSSETUP','DialogType','SL','BlockSet','RTICANMM','SlaveProcessor','CAN')), CANMMProperties=struct('cannedy',struct('data',struct('options',struct('controllername','RCM_Harness','controllernameautomatic',0,'loglevel','0','checkrealtime',0,'checkchangebaudrate',0,'sampletime','1.000','CANControllerStatus',1,'NumberofStuffErr',1,'NumberofFormErr',1,'NumberofAckErr',0,'NumberofBit0Err',0,'NumberofsuccrecRX',1,'Numberofsuccsent',1,'NumberofBit1Err',0,'NumberofCRCErr',1,'NumberoflostRX',1,'Busoff',0,'Busload',0,'OperationPending',0,'TxRetryCount',3,'addtrcexclusion',true,'cannavigator',struct('checkmonitoring',0,'checkinternmonitoring',0),'show_usrtrc',0,'use_usrtrc',0,'checkchangebaudrateFD',0,'errorframegeneration',0,'efgenabled',1),'modelroot','C:\GitDev\Yunli\FordMachE\HIL-Operation\src_cm4sl','generalsettings',struct('setupdata',struct('board','DS2671','boardno',1,'channelno',1,'Type','STD','transceiver',['ISO 11898-2 HIGH SPEED CAN'],'busconfig',[],'feedthrough','false','resistance',struct('r120',1,'roff',0,'r16',1,'r10',0),'baudrate','500','Frequency',[24 36],'samplemode',1,'commChannelTJA1041',6,'config',struct('standard',1,'advanced',0,'register',struct('btr0','0xC0','btr1','0x6F','sp','70','sjw','v','tseg1','15','tseg2','6','brp','0','smpl','0','btr0_36','0x1','btr1_36','0x2D','sp_36','83','sjw_36','0','tseg1_36','12','tseg2_36','2','brp_36','1','smpl_36','0','btr0_64','0x3','btr1_64','0x2B','sp_64','81','sjw_64','0','tseg1_64','11','tseg2_64','2','brp_64','3','smpl_64','0')),'channelcfg',struct('INTENDISABLE','CAN_INT_DISABLE','intenable',0),'SETUPID','RTICANMM_RCM_Harness_ID','CONTROLLER_ID','CANMM_CTL_SETUP_RCM_Harness','mainblock_includefile','RTICANMM_SETUP_RCM_Harness','canfdenable',0,'canfdboardselected',1,'slotno',1,'moduletype','DS4342','baudrateFD','2000','samplePoint','80','samplePointFD','80','termination','TERMINATION_ON'),'filesettings',struct('destfolder',struct('Name','RTICANMM_FILES','Check',1),'buildfolder',struct('Name','.','Check',1))),'advanced',struct('options',ones(1,100)),'partialnetdata',struct('switchedon',0,'format','STD','idmask',['XXXXX XXXXXXXX XXXXXXXX XXXXXXXX'],'idcode','0','idfilter','0','datamaskused',0,'datalength','0','datamask','0x0000000000000000','partialnetworkenable',0)),'blk',['HIL_MachE_CM10/Vehicle Under Test/Vehicle/MachE CAN/RTICANMM' char(10) 'RCM_Harness'],'allgeneratedfiles',{{'C:\GitDev\Yunli\FordMachE\HIL-Operation\src_cm4sl\RTICANMM_FILES\RTICANMM_SETUP_RCM_ECU.c','C:\GitDev\Yunli\FordMachE\HIL-Operation\src_cm4sl\RTICANMM_FILES\RTICANMM_SETUP_RCM_ECU.h','C:\GitDev\Yunli\FordMachE\HIL-Operation\src_cm4sl\RTICANMM_FILES\RTICANMM_SETUP_RCM_Harness.c','C:\GitDev\Yunli\FordMachE\HIL-Operation\src_cm4sl\RTICANMM_FILES\RTICANMM_SETUP_RCM_Harness.h','c:\gitdev\yunli\fordmache\hil-operation\src_cm4sl\rticanmm_files\rticanmm_setup_rcm_ecu.mexw64','c:\gitdev\yunli\fordmache\hil-operation\src_cm4sl\rticanmm_files\rticanmm_setup_rcm_harness.mexw64'}},'ismp',false,'BlockDataVersion','0.9.0','recreate',0,'CANnedyTag','RCM_Harness'),'CANnedynew',0,'CANnedySettings','RCM_Harness','GeneratedFiles',{{'C:\GitDev\Yunli\FordMachE\HIL-Operation\src_cm4sl\RTICANMM_FILES\RTICANMM_SETUP_RCM_ECU.c','C:\GitDev\Yunli\FordMachE\HIL-Operation\src_cm4sl\RTICANMM_FILES\RTICANMM_SETUP_RCM_ECU.h','C:\GitDev\Yunli\FordMachE\HIL-Operation\src_cm4sl\RTICANMM_FILES\RTICANMM_SETUP_RCM_Harness.c','C:\GitDev\Yunli\FordMachE\HIL-Operation\src_cm4sl\RTICANMM_FILES\RTICANMM_SETUP_RCM_Harness.h','c:\gitdev\yunli\fordmache\hil-operation\src_cm4sl\rticanmm_files\rticanmm_setup_rcm_ecu.mexw64','c:\gitdev\yunli\fordmache\hil-operation\src_cm4sl\rticanmm_files\rticanmm_setup_rcm_harness.mexw64'}},'SFCN','RTICANMM_SETUP_RCM_Harness.c','HostService',struct('Tags',struct('DATA','RTICANMM_MonitorData','TimeStampGlobal','RTICANMM_MonitoringTimeStamp','TimeStampGlobalEnable','RTICANMM_MonitoringTimeStampEnable','Enable','CANMMMonitor_RCM_Harness','TimeStamp','MonitoringTimeStamp_RCM_Harness'),'DATA',struct('Length',18),'Info',struct('Desc',{'ID','Service','Data1','Data2','Data3','Data4','Data5','Data6','Data7','Data8','Data9','Data10','Data11','Data12','Data13','Data14','Data15','Data16'}),'Names',struct('TimeStampGlobal','TimeStamp','TimeStampGlobalEnable','TimeStamp_Enable','Enable','Monitoring_Enable','TimeStamp','Monitoring_TimeStamp'),'ChannelID',3)), CANMMType=CANnedySetup, CANMMFolder=C:\CM_Projects\UA_cave\CM13_proj\src_cm4dspace_realsim, CANMMDestFolder=RTICANMM_FILES, CANMMSettings=RCM_Harness, CANMMSFcn=RTICANMM_SETUP_RCM_Harness, CANMMBoard=DS2671, CANMMBoardNum=1, CANMMChannel=1}
      settings: AttributesFormatString=%<CANMMSettings>  CopyFcn=rticanmm_blockfcn('CopyFcn', 'CANnedySetup', gcb)  DeleteFcn=rticanmm_blockfcn('DeleteFcn', 'CANnedySetup', gcb)  ModelCloseFcn=rticanmm_blockfcn('ModelCloseFcn', 'CANnedySetup', gcb)  NameChangeFcn=rticanmm_blockfcn('NameChangeFcn', 'CANnedySetup', gcb)  OpenFcn=try, rticanmm_setup_gui('create',gcb); ; catch,errordlg({lasterr, '','Please check your RTI installation.'},['Error: ' upper(bdroot)], 'replace'); end  MoveFcn=rticanmm_blockfcn('MoveFcn', 'CANnedySetup', gcb)
      mask Help: eval('rticanmm_quickstart(''create'', gcb);', 'disp(lasterr);')
      mask Display:
      | disp('RTI CAN\nMultiMessage\nControllerSetup')
      | 
      | port_label('input', 1 , 'Variation')
      | port_label('input', 2 , 'Reset')
      | port_label('output', 1, 'Status')
      | port_label('output', 2, 'Stuff errors')
      | port_label('output', 3, 'Format errors')
      | port_label('output', 4, 'CRC errors')
      | port_label('output', 5, 'RX lost')
      | port_label('output', 6, 'RX ok')
      | port_label('output', 7, 'TX ok')
  RTICANMM RCM_Harness1 : dsmpblib/Data Outport  Priority=-10000  Commented=on
      settings: SourceProductName=dSPACE Model Interface Package for Simulink (MIPS)
  Reset@RTICANMM ControllerSetup1 : Constant  Value=0  OutDataTypeStr=boolean
  Reset@RTICANMM ControllerSetup2 : Constant  Value=0  OutDataTypeStr=boolean
  Reset@RTICANMM ControllerSetup3 : Constant  Value=0  OutDataTypeStr=boolean
  Subsystem : Subsystem
  Terminator{,2..4} (4 alike) : Terminator  Commented=on
  Terminator1 : Terminator
  User2RTICANMM MainBlock1 : Subsystem
      mask Display: disp('Mapping\nto RTICANMM')
  User2RTICANMM MainBlock2 : Subsystem  Commented=on
      mask Display: disp('Mapping\nto RTICANMM')
  Variation@RTICANMM ControllerSetup1 : Constant  OutDataTypeStr=uint8
  Variation@RTICANMM ControllerSetup2 : Constant  OutDataTypeStr=uint8
  Variation@RTICANMM ControllerSetup3 : Constant  OutDataTypeStr=uint8
  buscreator : BusCreator  Inputs=3
  buscreator1 : BusCreator  Inputs=2
  gain : Gain
  gain1 : Gain
  gain2 : Gain
  Steering_ang_deg : Outport
  wires:
  Gain/1 -> Terminator/1  "GearPos_D_Actl"
  Gain1/1 -> Terminator2/1  "BattTrac_I2_Actl"
  Gain2/1 -> Terminator3/1  "BattTrac_U2_Actl"
  Reset@RTICANMM ControllerSetup1/1 -> RTICANMM RCM_ECU/2(Reset)
  Variation@RTICANMM ControllerSetup1/1 -> RTICANMM RCM_ECU/1(VariationInput)
  Variation@RTICANMM ControllerSetup2/1 -> RTICANMM RCM_Harness/1(VariationInput)
  Reset@RTICANMM ControllerSetup2/1 -> RTICANMM RCM_Harness/2(Reset)
  Constant/1 -> RTICANMM Gateway/1(Enable)
  RTICANMM MainBlock/1(RX_Data) -> Bus Selector1/1
  Bus Selector1/3 -> Subsystem/5(A_z), buscreator/3  "<VehVert2_A_Actl>"
  Bus Selector1/5 -> Subsystem/4(A_y), buscreator/2  "<VehLong2_A_Actl>"
  Bus Selector1/7 -> Subsystem/3(A_x), buscreator/1  "<VehLat2_A_Actl>"
  Bus Selector1/13 -> Subsystem/2(Yaw), buscreator1/2  "<VehYaw_W_Actl>"
  Bus Selector1/14 -> Subsystem/1(Roll), buscreator1/1  "<VehRol_W_Actl>"
  User2RTICANMM MainBlock1/1(out) -> RTICANMM MainBlock1/1(TXData)
  Bus Selector1/12 -> Bus Creator/4  "<VehRollYawW_No_Cs>"
  Bus Selector1/11 -> Bus Creator/3  "<VehRollYaw_No_Cnt>"
  Bus Selector1/10 -> Bus Creator/2  "<VehRolWActl_D_Qf>"
  Bus Selector1/9 -> Bus Creator/1  "<VehYawWActl_D_Qf>"
  Bus Creator/1 -> User2RTICANMM MainBlock1/2(Yaw)
  Bus Selector1/8 -> Bus Creator1/8  "<VehLatAActl_D_Qf>"
  Bus Selector1/6 -> Bus Creator1/6  "<VehLongAActl_D_Qf>"
  Bus Selector1/4 -> Bus Creator1/4  "<VehVertAActl_D_Qf>"
  Bus Selector1/2 -> Bus Creator1/2  "<VehLatLongVertA_No_Cs>"
  Bus Selector1/1 -> Bus Creator1/1  "<VehLatLongVert_No_Cnt>"
  Bus Creator1/1 -> User2RTICANMM MainBlock1/1("Accel_Data ")
  Subsystem/1(Accel_Data_out) -> Multiport Switch/3
  Bus Selector2/1 -> gain/1  "<VehLat2_A_Actl>"
  Bus Selector2/2 -> gain1/1  "<VehLong2_A_Actl>"
  Bus Selector2/3 -> gain2/1  "<VehVert2_A_Actl>"
  Subsystem/2(Yaw_Data_out) -> Multiport Switch1/3
  Bus Selector3/1 -> Gain5/1  "<VehRol_W_Actl>"
  Bus Selector3/2 -> Gain4/1  "<VehYaw_W_Actl>"
  Multiport Switch/1 -> Bus Selector2/1
  buscreator/1 -> Multiport Switch/2  "Accel_Data"
  Constant1/1 -> [RCM_Bypass], Multiport Switch/1
  Multiport Switch1/1 -> Bus Selector3/1
  buscreator1/1 -> Multiport Switch1/2  "Yaw_Data"
  [RCM_Bypass] -> Multiport Switch1/1
  RTICANMM MainBlock1/1(RX_Data) -> Bus Selector4/1
  Bus Selector4/1 -> Gain3/1  "<StePinRelInit_An_Sns>"
  RTICANMM RCM_Harness/1(BUS_STATE) -> Terminator1/1
  Gain3/1 -> Steering_ang_deg/1  "StePinRelInit_An_Sns"
  Gain4/1 -> Bus Creator/5  "VehYaw_W_Actl"
  Gain5/1 -> Bus Creator/6  "VehRol_W_Actl"
  gain/1 -> Bus Creator1/7  "VehLat2_A_Actl"
  gain1/1 -> Bus Creator1/5  "VehLong2_A_Actl"
  gain2/1 -> Bus Creator1/3  "VehVert2_A_Actl"
  Variation@RTICANMM ControllerSetup3/1 -> RTICANMM MachE_HS1/1(VariationInput)
  Reset@RTICANMM ControllerSetup3/1 -> RTICANMM MachE_HS1/2(Reset)
  Bus Selector/1 -> Gain2/1  "<BattTrac_U2_Actl>"
  Bus Selector/2 -> Gain1/1  "<BattTrac_I2_Actl>"
  Bus Selector/3 -> Gain/1  "<GearPos_D_Actl>"
  Gain6/1 -> Terminator4/1  "GearLvr_D_Actl"
  Bus Selector/4 -> Gain6/1  "<GearLvr_D_ActlDrv>"
  User2RTICANMM MainBlock2/1(out) -> RTICANMM MainBlock2/1(TXData)

== system Copy_of_CM13_2024a_MachE_for_UA_HIL/CarMaker_new/IPG Vehicle/PowerTrain ==
  note: When replacing the entire powertrain,
      | be sure to disable the IPG powertrain model by using the powertrain
      | model 'Model Manager off' in the vehicle GUI.
  note: <Your model here>
  VehicleSimulationType : Inport
  Sync_In : Inport  Port=2
  Vhcl.Wheel.PT : Inport  Port=3
  VhclCtrl.PT : Inport  Port=4
  VhclCtrl.PTUpd : Inport  Port=5
  BusCreator1 : BusCreator  Inputs=42
  Demux1 : Demux  Outputs=42
      settings: DisplayOption=none
  PowerTrain : S-Function  FunctionName=CM_Sfun  Parameters='PowerTrain'  SFunctionDeploymentMode=off  EnableBusSupport=off
  PowerTrainUpd : S-Function  FunctionName=CM_Sfun  Parameters='PowerTrainUpd'  SFunctionDeploymentMode=off  EnableBusSupport=off
  Switch : Switch  Criteria=u2 > Threshold  SaturateOnIntegerOverflow=off  InputSameDT=off
  Sync_Out : Outport  VectorParamsAs1DForOutWhenUnconnected=off
  wires:
  BusCreator1/1 -> Switch/3
  Demux1/42 -> BusCreator1/42  "PT IF WRR Trq_BrakeReg_max"
  Demux1/41 -> BusCreator1/41  "PT IF WRR Trq_BrakeReg"
  Demux1/40 -> BusCreator1/40  "PT IF WRR Trq_Supp2WC"
  Demux1/39 -> BusCreator1/39  "PT IF WRR Trq_Drive"
  Demux1/38 -> BusCreator1/38  "PT IF WRR Trq_B2W"
  Demux1/37 -> BusCreator1/37  "PT IF WRR rotv"
  Demux1/36 -> BusCreator1/36  "PT IF WRR rot"
  Demux1/35 -> BusCreator1/35  "PT IF WRL Trq_BrakeReg_max"
  Demux1/34 -> BusCreator1/34  "PT IF WRL Trq_BrakeReg"
  Demux1/33 -> BusCreator1/33  "PT IF WRL Trq_Supp2WC"
  Demux1/32 -> BusCreator1/32  "PT IF WRL Trq_Drive"
  Demux1/31 -> BusCreator1/31  "PT IF WRL Trq_B2W"
  Demux1/30 -> BusCreator1/30  "PT IF WRL rotv"
  Demux1/29 -> BusCreator1/29  "PT IF WRL rot"
  Demux1/28 -> BusCreator1/28  "PT IF WFR Trq_BrakeReg_max"
  Demux1/27 -> BusCreator1/27  "PT IF WFR Trq_BrakeReg"
  Demux1/26 -> BusCreator1/26  "PT IF WFR Trq_Supp2WC"
  Demux1/25 -> BusCreator1/25  "PT IF WFR Trq_Drive"
  Demux1/24 -> BusCreator1/24  "PT IF WFR Trq_B2W"
  Demux1/23 -> BusCreator1/23  "PT IF WFR rotv"
  Demux1/22 -> BusCreator1/22  "PT IF WFR rot"
  Demux1/21 -> BusCreator1/21  "PT IF WFL Trq_BrakeReg_max"
  Demux1/20 -> BusCreator1/20  "PT IF WFL Trq_BrakeReg"
  Demux1/19 -> BusCreator1/19  "PT IF WFL Trq_Supp2WC"
  Demux1/18 -> BusCreator1/18  "PT IF WFL Trq_Drive"
  Demux1/17 -> BusCreator1/17  "PT IF WFL Trq_B2W"
  Demux1/16 -> BusCreator1/16  "PT IF WFL rotv"
  Demux1/15 -> BusCreator1/15  "PT IF WFL rot"
  Demux1/14 -> BusCreator1/14  "PT IF DL_iDiff_mean"
  Demux1/13 -> BusCreator1/13  "PT IF Trq_Supp2BdyEng y"
  Demux1/12 -> BusCreator1/12  "PT IF Trq_Supp2BdyEng x"
  Demux1/11 -> BusCreator1/11  "PT IF Trq_Supp2Bdy1B z"
  Demux1/10 -> BusCreator1/10  "PT IF Trq_Supp2Bdy1B y"
  Demux1/9 -> BusCreator1/9  "PT IF Trq_Supp2Bdy1B x"
  Demux1/8 -> BusCreator1/8  "PT IF Trq_Supp2Bdy1 z"
  Demux1/7 -> BusCreator1/7  "PT IF Trq_Supp2Bdy1 y"
  Demux1/6 -> BusCreator1/6  "PT IF Trq_Supp2Bdy1 x"
  Demux1/5 -> BusCreator1/5  "PT IF Engine_rotv"
  Demux1/4 -> BusCreator1/4  "PT IF GearNo"
  Demux1/3 -> BusCreator1/3  "PT IF OperationError"
  Demux1/2 -> BusCreator1/2  "PT IF OperationState"
  Demux1/1 -> BusCreator1/1  "PT IF Ignition"
  Sync_In/1 -> PowerTrain/1
  PowerTrain/2 -> Demux1/1
  PowerTrainUpd/1 -> Sync_Out/1
  PowerTrain/1 -> PowerTrainUpd/1  "Sync"
  VhclCtrl.PT/1 -> PowerTrain/3
  Vhcl.Wheel.PT/1 -> PowerTrain/2
  VehicleSimulationType/1 -> Switch/2
  VhclCtrl.PTUpd/1 -> Switch/1
  Switch/1 -> PowerTrainUpd/2

== system Copy_of_CM13_2024a_MachE_for_UA_HIL/CarMaker_new/IPG Vehicle/Rototest UDP RX ExternalMode ==
  RT Dyno UDP Rx : dsmpblib/Data Inport  Priority=10000
      settings: SourceProductName=dSPACE Model Interface Package for Simulink (MIPS)
  RT Dyno UDP Tx_In : dsmpblib/Data Inport  Priority=10000
      settings: SourceProductName=dSPACE Model Interface Package for Simulink (MIPS)
  RT External Control : dsmpblib/Data Inport  Priority=10000
      settings: SourceProductName=dSPACE Model Interface Package for Simulink (MIPS)
  Terminator{2..8} (7 alike) : Terminator
  Data Vector : Outport
  wires:
  RT Dyno UDP Rx/1 -> Data Vector/1
  RT Dyno UDP Rx/2 -> Terminator2/1
  RT Dyno UDP Rx/3 -> Terminator3/1
  RT Dyno UDP Rx/4 -> Terminator4/1
  RT Dyno UDP Rx/5 -> Terminator5/1
  RT Dyno UDP Tx_In/2 -> Terminator8/1
  RT Dyno UDP Tx_In/1 -> Terminator7/1
  RT External Control/1 -> Terminator6/1

== system Copy_of_CM13_2024a_MachE_for_UA_HIL/CarMaker_new/IPG Vehicle/Rototest UDP TX ExternalMode ==
  Rototest_UDP_TX : Inport
  Cast : DataTypeConversion  SaturateOnIntegerOverflow=off  RndMeth=Floor
  Constant : Constant
  RT Dyno UDP Tx_Out : dsmpblib/Data Outport  Priority=-10000
      settings: SourceProductName=dSPACE Model Interface Package for Simulink (MIPS)
  wires:
  Rototest_UDP_TX/1 -> RT Dyno UDP Tx_Out/1
  Constant/1 -> Cast/1
  Cast/1 -> RT Dyno UDP Tx_Out/2
